simulink model "ACC2"  (R2023b)
settings: Solver=FixedStepAuto  StartTime=0.0  StopTime=inf  FixedStep=0.01  RelTol=1e-3
InitFcn:
  | params
libraries: arduinolib x9, arduinosensorlib x1
settings Model: ExtModeTrigDuration=2  Creator=SJ  LastModifiedBy=tkdle
settings SolverCC: AutoInsertRateTranBlk=on
settings OptimizationCC: EnhancedBackFolding=on  PassReuseOutputArgsAs=Individual arguments  ZeroExternalMemoryAtStartup=off  ZeroInternalMemoryAtStartup=off  MaxStackSize=64  OptimizeBlockOrder=speed  DifferentSizesBufferReuse=on  OptimizationCustomize=off  EfficientTunableParamExpr=on
settings DebuggingCC: MultiTaskRateTransMsg=warning  ParameterTunabilityLossMsg=error
settings HardwareCC: ProdBitPerInt=16  ProdBitPerPointer=16  ProdBitPerSizeT=16  ProdBitPerPtrDiffT=16  ProdLargestAtomicFloat=None  ProdWordSize=8  ProdHWDeviceType=Atmel->AVR
settings SFSimCC: MATLABDynamicMemAlloc=off
settings RTWCC: Description=Embedded Coder  SystemTargetFile=ert.tlc  HardwareBoard=Arduino Mega 2560  TemplateMakefile=ert_default_tmf  Toolchain=Arduino AVR  BuildConfiguration=Faster Runs
settings CodeAppCC: ForceParamTrailComments=on  IgnoreCustomStorageClasses=off  OperatorAnnotations=on  SimulinkDataObjDesc=on  SFDataObjDesc=on  InsertBlockDesc=on
settings ERTTargetCC: SupportContinuousTime=on  SupportVariableSizeSignals=on  ExtModeTransport=3  ExtModeStaticAlloc=on  ExtModeAutomaticAllocSize=off  ExtModeStaticAllocSize=2048  ExtModeMexFile=ext_xcp  ExtModeIntrfLevel=Level2 - Open

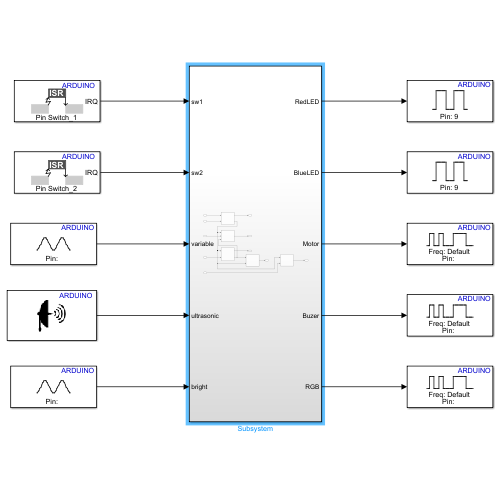
[thumbnail: Simulink's stored preview of the top-level diagram]
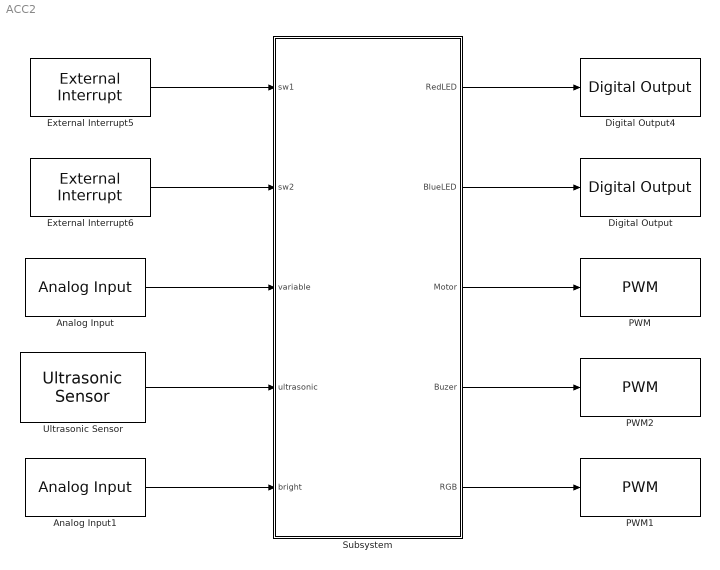
== system ACC2 ==
  Analog Input : arduinolib/Analog Input  pinNumber=Potentiometer  ReadResultsOnly=off  ConversionTriggerSource=Software  ExternalTriggerType=uint32( 0 )  OutputDataType=uint16  EnableConversionCompleteNotify=off  EnableOuputStatus=off  SampleTime=-1  blockPlatform=arduino
  Analog Input1 : arduinolib/Analog Input  pinNumber=Bright  ReadResultsOnly=off  ConversionTriggerSource=Software  ExternalTriggerType=uint32( 0 )  OutputDataType=uint16  EnableConversionCompleteNotify=off  EnableOuputStatus=off  SampleTime=-1  blockPlatform=arduino
  Digital Output : arduinolib/Digital Output  pinNumber=Blue_LED  Direction=output  blockPlatform=arduino
  Digital Output4 : arduinolib/Digital Output  pinNumber=Red_LED  Direction=output  blockPlatform=arduino
  External Interrupt5 : arduinolib/External Interrupt  Pin=Switch_1  PullUp=off  Mode=FALLING  InterruptSimulationInput=off
  External Interrupt6 : arduinolib/External Interrupt  Pin=Switch_2  PullUp=off  Mode=FALLING  InterruptSimulationInput=off
  PWM : arduinolib/PWM  pinNumber=Motor  frequencyType=Default  desiredFrequency=490.2  achievableFrequency=490.2
  PWM1 : arduinolib/PWM  pinNumber=RGB_LED  frequencyType=Default  desiredFrequency=490.2  achievableFrequency=490.2
  PWM2 : arduinolib/PWM  pinNumber=Buzzer  frequencyType=Default  desiredFrequency=490.2  achievableFrequency=490.2
  Subsystem : Subsystem
  Ultrasonic Sensor : arduinosensorlib/Ultrasonic Sensor  NumSignalPins=2  TrigPin=US_trigger  EchoPin=US_echo  SignalPin=3  SampleTime_=0.1  blockPlatform=ARDUINO
  wires:
  External Interrupt5/1 -> Subsystem/1(sw1)
  Subsystem/3(Motor) -> PWM/1
  Subsystem/4(Buzer) -> PWM2/1
  External Interrupt6/1 -> Subsystem/2(sw2)
  Subsystem/2(BlueLED) -> Digital Output/1
  Analog Input/1 -> Subsystem/3(variable)
  Ultrasonic Sensor/1 -> Subsystem/4(ultrasonic)
  Subsystem/1(RedLED) -> Digital Output4/1
  Analog Input1/1 -> Subsystem/5(bright)
  Subsystem/5(RGB) -> PWM1/1

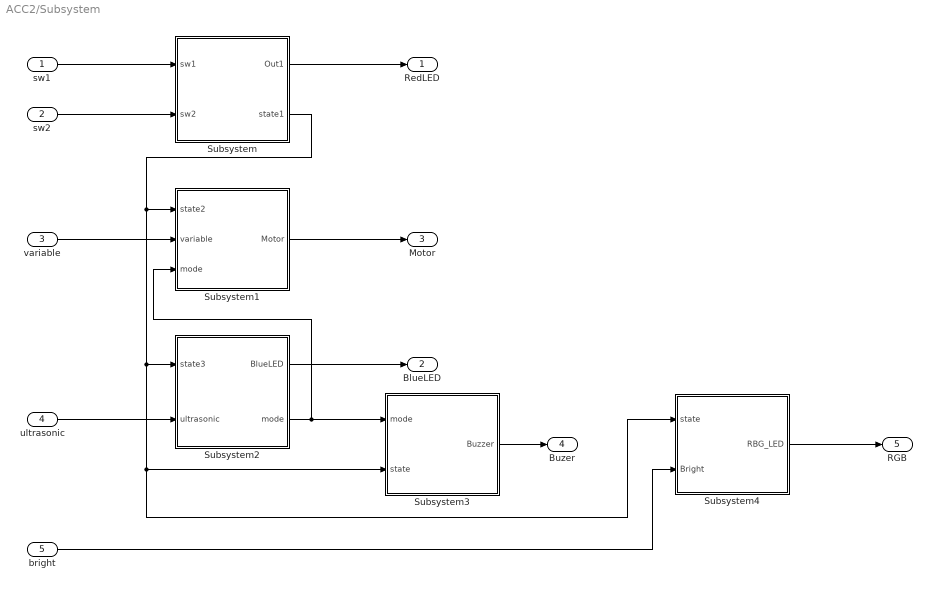
== system ACC2/Subsystem ==
  sw1 : Inport
  sw2 : Inport  Port=2
  variable : Inport  Port=3
  ultrasonic : Inport  Port=4
  bright : Inport  Port=5
  Subsystem : Subsystem
  Subsystem1 : Subsystem
  Subsystem2 : Subsystem
  Subsystem3 : Subsystem
  Subsystem4 : Subsystem
  RedLED : Outport
  BlueLED : Outport  Port=2
  Motor : Outport  Port=3
  Buzer : Outport  Port=4
  RGB : Outport  Port=5
  wires:
  sw1/1 -> Subsystem/1(sw1)
  sw2/1 -> Subsystem/2(sw2)
  Subsystem/1(Out1) -> RedLED/1
  Subsystem/2(state1) -> Subsystem1/1(state2), Subsystem2/1(state3), Subsystem4/1(state), Subsystem3/2(state)
  variable/1 -> Subsystem1/2(variable)
  ultrasonic/1 -> Subsystem2/2(ultrasonic)
  Subsystem2/1(BlueLED) -> BlueLED/1
  Subsystem1/1(Motor) -> Motor/1
  Subsystem2/2(mode) -> Subsystem3/1(mode), Subsystem1/3(mode)
  Subsystem3/1(Buzzer) -> Buzer/1
  bright/1 -> Subsystem4/2(Bright)
  Subsystem4/1(RBG_LED) -> RGB/1

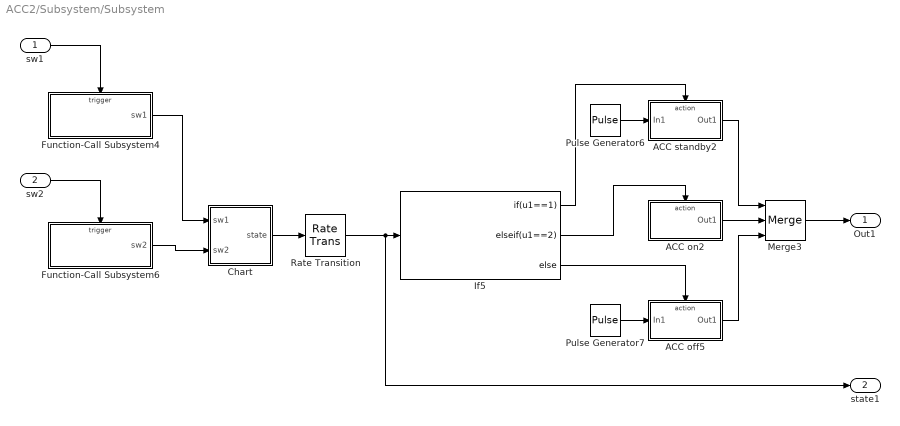
== system ACC2/Subsystem/Subsystem ==
  sw1 : Inport
  sw2 : Inport  Port=2
  ACC off5 : Subsystem  TreatAsAtomicUnit=on
  ACC on2 : Subsystem  TreatAsAtomicUnit=on
  ACC standby2 : Subsystem  TreatAsAtomicUnit=on
  Chart : Stateflow chart  TreatAsAtomicUnit=on
  Function-Call Subsystem4 : Subsystem  TreatAsAtomicUnit=on
  Function-Call Subsystem6 : Subsystem  TreatAsAtomicUnit=on
  If5 : If  IfExpression=u1==1  ElseIfExpressions=u1==2
  Merge3 : Merge  Inputs=3
  Pulse Generator6 : DiscretePulseGenerator  PulseType=Time based  Period=0.4  PulseWidth=50
  Pulse Generator7 : DiscretePulseGenerator  PulseType=Time based  PulseWidth=50
  Rate Transition : RateTransition  Deterministic=off  OutPortSampleTime=0.01
  Out1 : Outport
  state1 : Outport  Port=2
  wires:
  If5/2 -> ACC on2/Action
  Pulse Generator6/1 -> ACC standby2/1(In1)
  ACC standby2/1(Out1) -> Merge3/1
  sw2/1 -> Function-Call Subsystem6/Trigger
  sw1/1 -> Function-Call Subsystem4/Trigger
  If5/1 -> ACC standby2/Action
  ACC off5/1(Out1) -> Merge3/3
  ACC on2/1(Out1) -> Merge3/2
  Pulse Generator7/1 -> ACC off5/1(In1)
  Function-Call Subsystem6/1(sw2) -> Chart/2(sw2)
  Merge3/1 -> Out1/1
  If5/3 -> ACC off5/Action
  Chart/1(state) -> Rate Transition/1
  Function-Call Subsystem4/1(sw1) -> Chart/1(sw1)
  Rate Transition/1 -> state1/1, If5/1

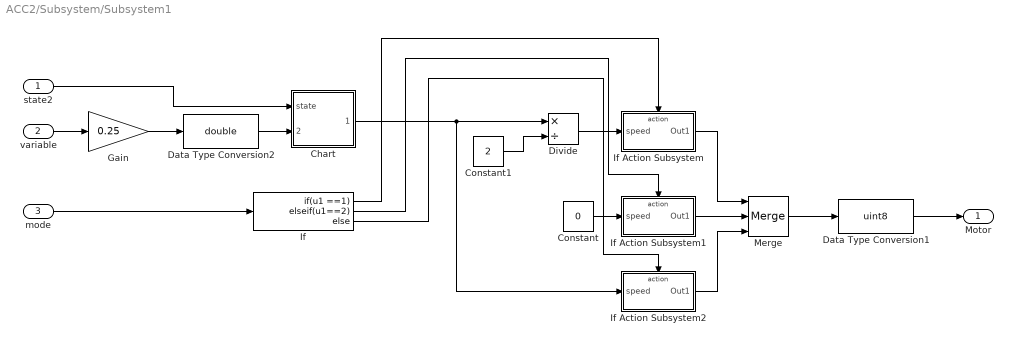
== system ACC2/Subsystem/Subsystem1 ==
  state2 : Inport
  variable : Inport  Port=2
  mode : Inport  Port=3
  Chart : Stateflow chart  TreatAsAtomicUnit=on
  Constant : Constant  Value=0
  Constant1 : Constant  Value=2
  Data Type Conversion1 : DataTypeConversion  OutDataTypeStr=uint8  SaturateOnIntegerOverflow=off  RndMeth=Floor
  Data Type Conversion2 : DataTypeConversion  OutDataTypeStr=double  SaturateOnIntegerOverflow=off  RndMeth=Floor
  Divide : Product  Inputs=*/
  Gain : Gain  Gain=0.25
  If : If  IfExpression=u1 ==1  ElseIfExpressions=u1==2
  If Action Subsystem : Subsystem  TreatAsAtomicUnit=on
  If Action Subsystem1 : Subsystem  TreatAsAtomicUnit=on
  If Action Subsystem2 : Subsystem  TreatAsAtomicUnit=on
  Merge : Merge  Inputs=3
  Motor : Outport
  wires:
  Data Type Conversion2/1 -> Chart/2(variable)
  Data Type Conversion1/1 -> Motor/1
  variable/1 -> Gain/1
  state2/1 -> Chart/1(state)
  Gain/1 -> Data Type Conversion2/1
  mode/1 -> If/1
  Merge/1 -> Data Type Conversion1/1
  Chart/1(speed) -> Divide/1, If Action Subsystem2/1(speed)
  If/1 -> If Action Subsystem/Action
  If/2 -> If Action Subsystem1/Action
  If/3 -> If Action Subsystem2/Action
  If Action Subsystem2/1(Out1) -> Merge/3
  Constant/1 -> If Action Subsystem1/1(speed)
  If Action Subsystem/1(Out1) -> Merge/1
  If Action Subsystem1/1(Out1) -> Merge/2
  Divide/1 -> If Action Subsystem/1(speed)
  Constant1/1 -> Divide/2

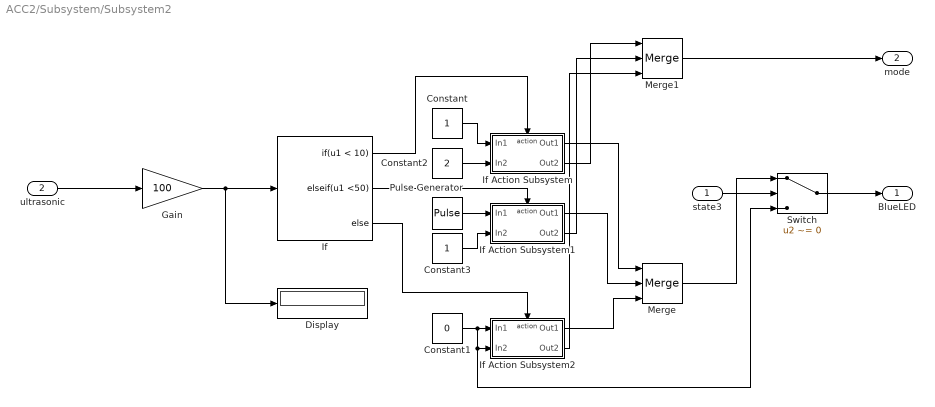
== system ACC2/Subsystem/Subsystem2 ==
  state3 : Inport
  ultrasonic : Inport  Port=2
  Constant : Constant
  Constant1 : Constant  Value=0
  Constant2 : Constant  Value=2
  Constant3 : Constant
  Display : Display
  Gain : Gain  Gain=100
  If : If  IfExpression=u1 < 10  ElseIfExpressions=u1 <50
  If Action Subsystem : Subsystem  TreatAsAtomicUnit=on
  If Action Subsystem1 : Subsystem  TreatAsAtomicUnit=on
  If Action Subsystem2 : Subsystem  TreatAsAtomicUnit=on
  Merge : Merge  Inputs=3
  Merge1 : Merge  Inputs=3
  Pulse Generator : DiscretePulseGenerator  PulseType=Time based  Period=0.4  PulseWidth=50
  Switch : Switch  Criteria=u2 ~= 0  SaturateOnIntegerOverflow=off  InputSameDT=off
  BlueLED : Outport
  mode : Outport  Port=2
  wires:
  Gain/1 -> If/1, Display/1
  If/1 -> If Action Subsystem/Action
  Constant/1 -> If Action Subsystem/1(In1)
  If Action Subsystem/1(Out1) -> Merge/1
  If/2 -> If Action Subsystem1/Action
  If/3 -> If Action Subsystem2/Action
  If Action Subsystem1/1(Out1) -> Merge/2
  If Action Subsystem2/1(Out1) -> Merge/3
  Constant1/1 -> If Action Subsystem2/2(In2), Switch/3, If Action Subsystem2/1(In1)
  Pulse Generator/1 -> If Action Subsystem1/1(In1)
  ultrasonic/1 -> Gain/1
  Merge/1 -> Switch/1
  state3/1 -> Switch/2
  Switch/1 -> BlueLED/1
  Constant2/1 -> If Action Subsystem/2(In2)
  Constant3/1 -> If Action Subsystem1/2(In2)
  If Action Subsystem/2(Out2) -> Merge1/1
  If Action Subsystem1/2(Out2) -> Merge1/2
  If Action Subsystem2/2(Out2) -> Merge1/3
  Merge1/1 -> mode/1

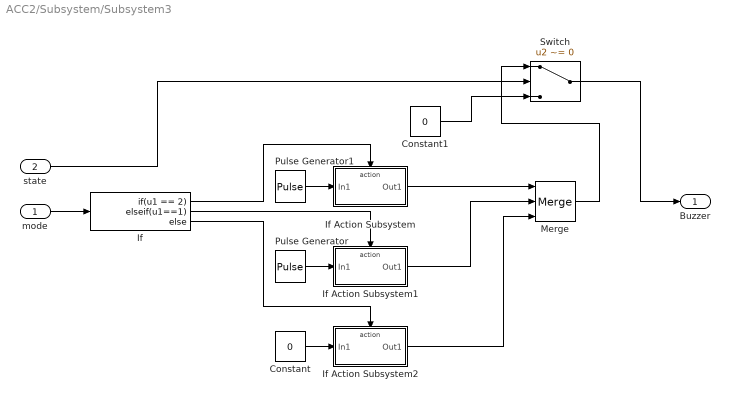
== system ACC2/Subsystem/Subsystem3 ==
  mode : Inport
  state : Inport  Port=2
  Constant : Constant  Value=0
  Constant1 : Constant  Value=0
  If : If  IfExpression=u1 == 2  ElseIfExpressions=u1==1
  If Action Subsystem : Subsystem  TreatAsAtomicUnit=on
  If Action Subsystem1 : Subsystem  TreatAsAtomicUnit=on
  If Action Subsystem2 : Subsystem  TreatAsAtomicUnit=on
  Merge : Merge  Inputs=3
  Pulse Generator : DiscretePulseGenerator  PulseType=Time based  PulseWidth=50
  Pulse Generator1 : DiscretePulseGenerator  PulseType=Time based  Period=0.4  PulseWidth=50
  Switch : Switch  Criteria=u2 ~= 0  SaturateOnIntegerOverflow=off  InputSameDT=off
  Buzzer : Outport
  wires:
  mode/1 -> If/1
  If Action Subsystem/1(Out1) -> Merge/1
  If Action Subsystem1/1(Out1) -> Merge/2
  If Action Subsystem2/1(Out1) -> Merge/3
  If/1 -> If Action Subsystem/Action
  If/2 -> If Action Subsystem1/Action
  If/3 -> If Action Subsystem2/Action
  Pulse Generator1/1 -> If Action Subsystem/1(In1)
  Pulse Generator/1 -> If Action Subsystem1/1(In1)
  Constant/1 -> If Action Subsystem2/1(In1)
  state/1 -> Switch/2
  Merge/1 -> Switch/1
  Constant1/1 -> Switch/3
  Switch/1 -> Buzzer/1

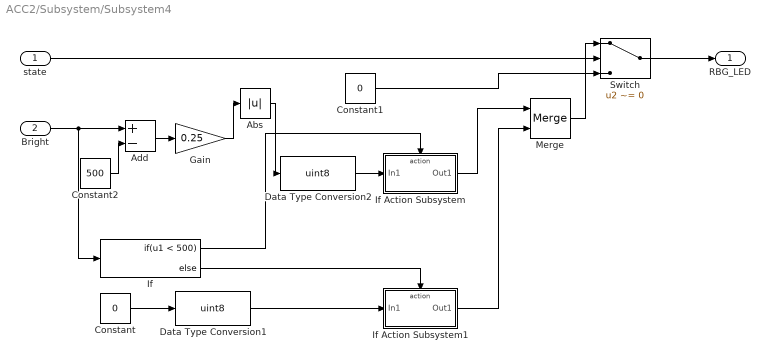
== system ACC2/Subsystem/Subsystem4 ==
  state : Inport
  Bright : Inport  Port=2
  Abs : Abs  SaturateOnIntegerOverflow=off
  Add : Sum  Inputs=+-  OutDataTypeStr=uint8
  Constant : Constant  Value=0
  Constant1 : Constant  Value=0
  Constant2 : Constant  Value=500
  Data Type Conversion1 : DataTypeConversion  OutDataTypeStr=uint8  SaturateOnIntegerOverflow=off  RndMeth=Floor
  Data Type Conversion2 : DataTypeConversion  OutDataTypeStr=uint8  SaturateOnIntegerOverflow=off  RndMeth=Floor
  Gain : Gain  Gain=0.25
  If : If  IfExpression=u1 < 500
  If Action Subsystem : Subsystem  TreatAsAtomicUnit=on
  If Action Subsystem1 : Subsystem  TreatAsAtomicUnit=on
  Merge : Merge
  Switch : Switch  Criteria=u2 ~= 0  SaturateOnIntegerOverflow=off  InputSameDT=off
  RBG_LED : Outport
  wires:
  Data Type Conversion1/1 -> If Action Subsystem1/1(In1)
  If/1 -> If Action Subsystem/Action
  If/2 -> If Action Subsystem1/Action
  Constant/1 -> Data Type Conversion1/1
  If Action Subsystem1/1(Out1) -> Merge/2
  If Action Subsystem/1(Out1) -> Merge/1
  Constant1/1 -> Switch/3
  Switch/1 -> RBG_LED/1
  state/1 -> Switch/2
  Merge/1 -> Switch/1
  Bright/1 -> Add/1, If/1
  Constant2/1 -> Add/2
  Gain/1 -> Abs/1
  Add/1 -> Gain/1
  Data Type Conversion2/1 -> If Action Subsystem/1(In1)
  Abs/1 -> Data Type Conversion2/1

== system ACC2/Subsystem/Subsystem/ACC off5 ==
  In1 : Inport
  Action Port : ActionPort  ActionPortLabel=else
  Out1 : Outport
  wires:
  In1/1 -> Out1/1

== system ACC2/Subsystem/Subsystem/ACC on2 ==
  Action Port : ActionPort  ActionPortLabel=elseif(u1==2)
  Constant : Constant
  Out1 : Outport
  wires:
  Constant/1 -> Out1/1

== system ACC2/Subsystem/Subsystem/ACC standby2 ==
  In1 : Inport
  ACC standby : ActionPort  ActionPortLabel=if(u1==1)
  Out1 : Outport
  wires:
  In1/1 -> Out1/1

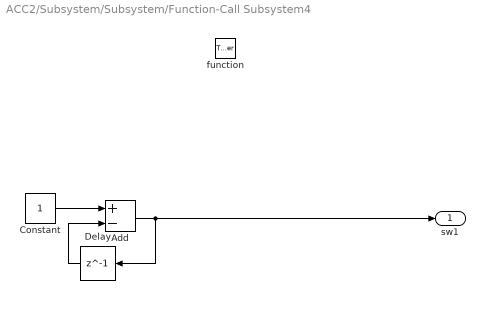
== system ACC2/Subsystem/Subsystem/Function-Call Subsystem4 ==
  function : TriggerPort  TriggerType=function-call  VariantControl=(inherit)
  Add : Sum  Inputs=+-
  Constant : Constant
  Delay : Delay  DelayLength=1
  sw1 : Outport
  wires:
  Add/1 -> sw1/1, Delay/1
  Delay/1 -> Add/2
  Constant/1 -> Add/1

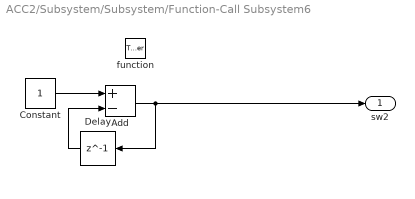
== system ACC2/Subsystem/Subsystem/Function-Call Subsystem6 ==
  function : TriggerPort  TriggerType=function-call  VariantControl=(inherit)
  Add : Sum  Inputs=+-
  Constant : Constant
  Delay : Delay  DelayLength=1
  sw2 : Outport
  wires:
  Constant/1 -> Add/1
  Delay/1 -> Add/2
  Add/1 -> sw2/1, Delay/1

== system ACC2/Subsystem/Subsystem1/If Action Subsystem ==
  speed : Inport
  Action Port : ActionPort  ActionPortLabel=if(u1 ==1)
  Out1 : Outport
  wires:
  speed/1 -> Out1/1

== system ACC2/Subsystem/Subsystem1/If Action Subsystem1 ==
  speed : Inport
  Action Port : ActionPort  ActionPortLabel=elseif(u1==2)
  Out1 : Outport
  wires:
  speed/1 -> Out1/1

== system ACC2/Subsystem/Subsystem1/If Action Subsystem2 ==
  speed : Inport
  Action Port : ActionPort  ActionPortLabel=else
  Out1 : Outport
  wires:
  speed/1 -> Out1/1

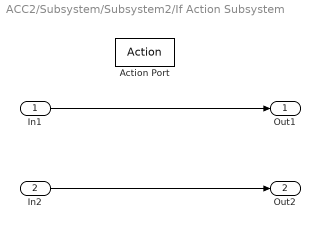
== system ACC2/Subsystem/Subsystem2/If Action Subsystem ==
  In1 : Inport
  In2 : Inport  Port=2
  Action Port : ActionPort  ActionPortLabel=if(u1 < 10)
  Out1 : Outport
  Out2 : Outport  Port=2
  wires:
  In1/1 -> Out1/1
  In2/1 -> Out2/1

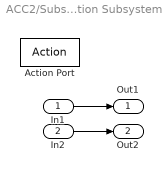
== system ACC2/Subsystem/Subsystem2/If Action Subsystem1 ==
  In1 : Inport
  In2 : Inport  Port=2
  Action Port : ActionPort  ActionPortLabel=elseif(u1 <50)
  Out1 : Outport
  Out2 : Outport  Port=2
  wires:
  In1/1 -> Out1/1
  In2/1 -> Out2/1

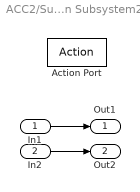
== system ACC2/Subsystem/Subsystem2/If Action Subsystem2 ==
  In1 : Inport
  In2 : Inport  Port=2
  Action Port : ActionPort  ActionPortLabel=else
  Out1 : Outport
  Out2 : Outport  Port=2
  wires:
  In1/1 -> Out1/1
  In2/1 -> Out2/1

== system ACC2/Subsystem/Subsystem3/If Action Subsystem ==
  In1 : Inport
  Action Port : ActionPort  ActionPortLabel=if(u1 == 2)
  Out1 : Outport
  wires:
  In1/1 -> Out1/1

== system ACC2/Subsystem/Subsystem3/If Action Subsystem1 ==
  In1 : Inport
  Action Port : ActionPort  ActionPortLabel=elseif(u1==1)
  Out1 : Outport
  wires:
  In1/1 -> Out1/1

== system ACC2/Subsystem/Subsystem3/If Action Subsystem2 ==
  In1 : Inport
  Action Port : ActionPort  ActionPortLabel=else
  Out1 : Outport
  wires:
  In1/1 -> Out1/1

== system ACC2/Subsystem/Subsystem4/If Action Subsystem ==
  In1 : Inport
  Action Port : ActionPort  ActionPortLabel=if(u1 < 500)
  Out1 : Outport
  wires:
  In1/1 -> Out1/1

== system ACC2/Subsystem/Subsystem4/If Action Subsystem1 ==
  In1 : Inport
  Action Port : ActionPort  ActionPortLabel=else
  Out1 : Outport
  wires:
  In1/1 -> Out1/1

== stateflow chart ACC2/Subsystem/Subsystem1/Chart ==
  state AccOff
    en,du:
    a=variable;
    speed=0;
  state AccStandby
    en,du:
    speed=a;
  state AccOn
    en,du:
    speed=variable;
  (default) -> AccOff
  AccOff -> AccStandby : [state==1]
  AccStandby -> AccOff [order 2] : [state==0]
  AccOn -> AccOff : [state==0]
  AccStandby -> AccOn [order 1] : [state==2]
  data: state input; variable input; a local; speed output

== stateflow chart ACC2/Subsystem/Subsystem/Chart ==
  state AccOff
    en,du:
    v1=sw1;
    v2=sw2;
    state=0;
  state AccStandby
    en,du:
    v1=sw1;
    v2=sw2;
    state=1;
  state AccOn
    en,du:
    v1=sw1;
    v2=sw2;
    state=2;
  (default) -> AccOff
  AccStandby -> AccOff [order 1] : [v2~=sw2]
  AccOff -> AccStandby : [v1~=sw1]
  AccOn -> AccOff [order 1] : [v1~=sw1]
  AccOn -> AccOff [order 2] : [v2~=sw2]
  AccStandby -> AccOn [order 2] : [v1~=sw1]
  data: sw1 input; state output; v1 local; v2 local; sw2 input
